simulink model "Joint_Space_Grav_Comp"  (R2020b)
settings: Solver=VariableStepAuto  StartTime=0.0  StopTime=10.0  RelTol=1e-3
values from neighbouring files (symbols this model uses):
  G = myRobot.G_Lagrangian    [hw6_main.m]    (also in joint_dynamics.m)
  Kd = diag([15,15,15])    [hw6_main.m]
  Kp = diag([20,20,20])    [hw6_main.m]
  qd = [0.1; 0.1; 0.15 ]    [hw6_main.m]
settings Model: Creator=nicol  LastModifiedBy=nicol

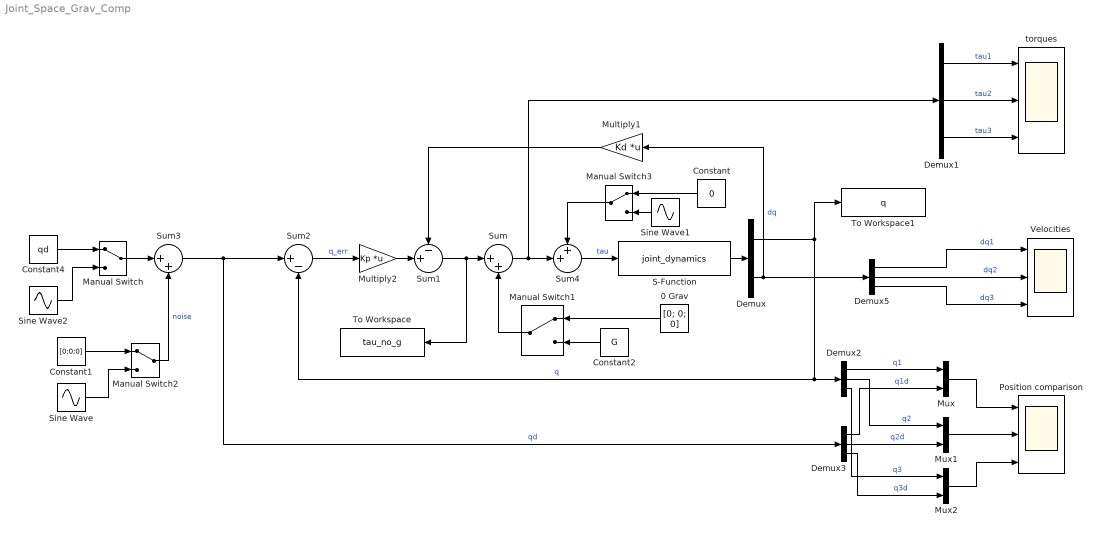
== system Joint_Space_Grav_Comp ==
  0 Grav : Constant  Value=[0; 0; 0]  VectorParams1D=off
  Constant : Constant  Value=0  VectorParams1D=off
  Constant1 : Constant  Value=[0;0;0]  VectorParams1D=off
  Constant2 : Constant  Value=G  VectorParams1D=off
  Constant4 : Constant  Value=qd  VectorParams1D=off
  Demux : Demux  Outputs=2
  Demux{1..3,5} (4 alike) : Demux  Outputs=3
  Manual Switch{,1..3} (4 alike) : ManualSwitch
  Multiply1 : Gain  Gain=Kd  Multiplication=Matrix(K*u)
  Multiply2 : Gain  Gain=Kp  Multiplication=Matrix(K*u)
  Mux : Mux  Inputs=2
  Mux1 : Mux  Inputs=2
  Mux2 : Mux  Inputs=2
  Position comparison : Scope  NumInputPorts=3
  S-Function : S-Function  FunctionName=joint_dynamics  Parameters=myRobot  SFunctionDeploymentMode=off  EnableBusSupport=off
  Sine Wave : Sin  Amplitude=0.1  SampleTime=0  VectorParams1D=off
  Sine Wave1 : Sin  Amplitude=0.1  Frequency=5  SampleTime=0  VectorParams1D=off
  Sine Wave2 : Sin  Amplitude=0.1  SampleTime=0
  Sum : Sum  Inputs=|++
  Sum1 : Sum  Inputs=-+|
  Sum2 : Sum  Inputs=|+-
  Sum3 : Sum  Inputs=|++
  Sum4 : Sum  Inputs=++|
  To Workspace : ToWorkspace  VariableName=tau_no_g  SaveFormat=Timeseries  SampleTime=-1
  To Workspace1 : ToWorkspace  VariableName=q  SaveFormat=Timeseries  SampleTime=-1
  Velocities : Scope  NumInputPorts=3
  torques : Scope  NumInputPorts=3
  wires:
  Sum/1 -> Sum4/2, Demux1/1
  Constant2/1 -> Manual Switch1/2
  Manual Switch1/1 -> Sum/2
  0 Grav/1 -> Manual Switch1/1
  Sum1/1 -> To Workspace/1, Sum/1
  Multiply1/1 -> Sum1/1
  Multiply2/1 -> Sum1/2
  Sum2/1 -> Multiply2/1  "q_err"
  Manual Switch2/1 -> Sum3/2  "noise"
  Constant1/1 -> Manual Switch2/1
  Sine Wave/1 -> Manual Switch2/2
  Demux1/2 -> torques/2  "tau2"
  Demux1/3 -> torques/3  "tau3"
  Demux1/1 -> torques/1  "tau1"
  Constant4/1 -> Manual Switch/1
  Sum3/1 -> Demux3/1, Sum2/1  "qd"
  S-Function/1 -> Demux/1
  Demux2/1 -> Mux/1  "q1"
  Demux3/1 -> Mux/2  "q1d"
  Demux2/2 -> Mux1/1  "q2"
  Demux3/2 -> Mux1/2  "q2d"
  Demux2/3 -> Mux2/1  "q3"
  Demux3/3 -> Mux2/2  "q3d"
  Mux/1 -> Position comparison/1
  Mux1/1 -> Position comparison/2
  Mux2/1 -> Position comparison/3
  Demux5/2 -> Velocities/2  "dq2"
  Demux5/1 -> Velocities/1  "dq1"
  Demux5/3 -> Velocities/3  "dq3"
  Demux/1 -> To Workspace1/1, Sum2/2, Demux2/1  "q"
  Demux/2 -> Multiply1/1, Demux5/1  "dq"
  Sum4/1 -> S-Function/1  "tau"
  Sine Wave1/1 -> Manual Switch3/2
  Manual Switch3/1 -> Sum4/1
  Constant/1 -> Manual Switch3/1
  Manual Switch/1 -> Sum3/1
  Sine Wave2/1 -> Manual Switch/2
